simulink model "AccelCtrl_ACC_test"  (R2019b)
settings: Solver=FixedStepAuto  StartTime=0.0  StopTime=inf  FixedStep=0.001  RelTol=1e-3  EnableMultiTasking=on
libraries: CarMaker4SL x42, simulink x3
(part 3 of 3)

== matlab function AccelCtrl_ACC_test/CarMaker/VehicleControl/AccelCtrl/ACC ECU/MATLAB Function ==
  data: v_f input; s_of_t output size=400; a_f input; dist input; v_ego input; a_ego input; KJ input; KT input; KDS input; KJV input; KTV input; KDSV input; speed_limit input; MAX_ACC input; MIN_ACC input; v_of_t output size=400; t_data output size=400; a_des output; cost_optimal output; SET_SPEED input
% clc
% clear all
% close all
% 
% 
% v_f = 10;
% a_f = 0;
% dist = 20;
% v_ego = 7;
% a_ego = 0;
% KJ = 1;
% KT = 1;
% KDS = 10;
% speed_limit= 20;
% MAX_ACC = 2;
% MIN_ACC = -3;
% 
% 
% [s_of_t, v_of_t,t_data] = acc_planning(v_f,a_f,dist,v_ego,a_ego,KJ,KT,KDS,speed_limit,MAX_ACC, MIN_ACC);
% 
% 
% figure
% plot(t_data,s_of_t,'-b')
% title("s of t")
% 
% figure
% plot(t_data,v_of_t,'-b')
% title("v of t")

function [s_of_t, v_of_t,t_data,a_des,cost_optimal] = acc_planning(v_f,a_f,dist,v_ego,a_ego,KJ,KT,KDS,KJV, KTV, KDSV,...
    speed_limit,MAX_ACC, MIN_ACC,SET_SPEED)

    DT = 1 ; % Delta T [s]
    MAXT = 5;% [s]
    MINT = 2; % [s]
    MINT_V = 2;
    MAXT_V = 10;
    
    
    DS = 0.5;
    DV = 0.5;
    
    D0 = 5;
    TTC = 3;
    s_of_t = zeros(200,1);
    v_of_t = zeros(200,1);
    t_data = zeros(200,1); 
    a_des = 0;
    cost_optimal = zeros(1,12);
    
    if dist > 100
        [cost_graph] = cal_velocity_control(MINT_V,DT,MAXT_V, SET_SPEED,DV,v_ego, a_ego,KJV, KTV, KDSV);
        [cost_optimal] = check_quantic_status(cost_graph,speed_limit, MAX_ACC, MIN_ACC);
        [s_of_t, v_of_t,t_data] = combination_quantic(cost_optimal);
        a_des = PID_control_a(v_of_t,v_ego);
   
        
    elseif dist > 0 && dist < 100
        
        cost_graph = cal_distance_control(MINT,DT,MAXT,v_f,a_f,dist,D0,TTC,DS,v_ego,a_ego,KJ,KT,KDS)
        cost_optimal = check_status(cost_graph,speed_limit, MAX_ACC, MIN_ACC);
        [s_of_t, v_of_t,t_data] = combination(cost_optimal);
        a_des = PID_control_a(v_of_t,v_ego);
    end
end


function a_des = PID_control_a(v_of_t,v_ego)
    a_des = 0.2 * (v_of_t(2) - v_ego);
end

function v_des = PID_control_v(v_of_t,v_ego)
    v_des = 1 * (v_of_t(2) - v_ego);
end


function v_f_t = cal_v_f_t(v_f, a_f, Ti)
    %calculate v_f of time.
    v_f_t = v_f + a_f * Ti;
end
    

function dist_t = cal_dist_t(dist,v_f,a_f,Ti)
    %calculate distance of time.
    dist_t = dist + v_f * Ti + 1/2 * a_f * Ti^2;
end


function [s_des] = cal_s_des(D0, TTC, v_f_t)
    %calculate desired s.
    s_des = D0 + TTC * v_f_t;
end


function [s_target] = cal_s_target(s_des,dist_t)
    %calculate s target.
    s_target = dist_t - s_des;
end

function [s_target_d] = cal_s_target_d(v_f_t, TTC, a_f)
    %calculate v_f of time.
    s_target_d = v_f_t - TTC * a_f;
end


function [s_target_dd] = cal_s_target_dd(a_f)
    s_target_dd = a_f;
end

function [cost_graph] = cal_distance_control(MINT,DT,MAXT,v_f,a_f,dist,D0,TTC,DS,v_ego,a_ego,KJ,KT,KDS)
    
    cost_graph = ones(400,12)* 500; 
    index = 1;
    for Ti = MINT : DT : MAXT
        v_f_t = cal_v_f_t(v_f, a_f, Ti);
        dist_t = cal_dist_t(dist,v_f,a_f,Ti);
        [s_des] = cal_s_des(D0, TTC, v_f_t);
        [s_target] = cal_s_target(s_des,dist_t);
        [s_target_d] = cal_s_target_d(v_f_t, TTC, a_f);
        [s_target_dd] = cal_s_target_dd(a_f);
        delta_s = 0.1 * s_target;
        
        for Si = (s_target - delta_s) : DS : (s_target + delta_s) 
            s0 = 0;
            v0 = v_ego;
            a0 = a_ego;
            se = Si;
            ve = s_target_d;
            ae = s_target_dd;
            [a0, a1, a2, a3, a4,a5] = quintic_polynomial(s0, ...
                v0, a0, se, ve, ae,Ti);
            %get the quintic polu parameters;
            [jerk] = cal_jerk(a3,a4,a5,Ti);
            cost_J = mean(abs(jerk));
            cost_T = Ti;
            cost_DS = sqrt((s_target - Si)^2);
            cost_total = KJ * cost_J + KT * cost_T + KDS * cost_DS;
            cost_graph(index,:) = [cost_total,Ti,Si,cost_J,cost_T,cost_DS,...
                a0, a1, a2, a3, a4, a5];
            
            index = index + 1;
        end
    end
    cost_graph = sortrows(cost_graph);
end

function [cost_graph] = cal_velocity_control(MINT_V,DT,MAXT_V, SET_SPEED,DV,v_ego, a_ego,KJV, KTV, KDSV)
    cost_graph = ones(400,11)* 500;    
    index = 1;
    delta_v = 0.1 * SET_SPEED;

    for Ti = MINT_V : DT : MAXT_V
        for Ve = SET_SPEED - delta_v : DV : SET_SPEED + delta_v 
            s0 = 0;
            v0 = v_ego;
            a0 = a_ego;
            ve = Ve;
            ae = 0;
            [a0, a1, a2, a3, a4] = quantic_polynomial(s0, ...
                v0, a0, ve, ae,Ti)
            [jerk] = cal_quantic_jerk(a3,a4,Ti);
            cost_J = mean(abs(jerk));
            cost_T = Ti;
            cost_DV = sqrt((SET_SPEED - Ve)^2);
            cost_total = KJV * cost_J + KTV * cost_T + KDSV * cost_DV;
            cost_graph(index,:) = [cost_total,Ti,Ve,cost_J,cost_T,cost_DV,...
                a0, a1, a2, a3, a4];

            index = index + 1;
        end
    end
        cost_graph = sortrows(cost_graph);
end


function [cost_optimal] = check_status(cost_graph,speed_limit, MAX_ACC, MIN_ACC)
    i = 1;
    COND = 1;
    cost_optimal = zeros(1,12);
    if isempty(cost_graph)
        cost_optimal=  zeros(1,12);
        fprintf("error in cost graph.");
        return;
    end
    
    
    
    while COND == 1
         
        vt = [];
        at = [];
        
        
        poly_para = cost_graph(i,7:12);
        a0 = poly_para(1); a1 = poly_para(2); a2 = poly_para(3); 
        a3 = poly_para(4); a4 = poly_para(5); a5 = poly_para(6);
        
        Te = cost_graph(i,2);
        
        
        
        for t = 0:0.5:Te
            vt = [vt, calc_first_derivative(a1,a2,a3,a4,a5,t)];
            at = [at, calc_second_derivative(a2,a3,a4,a5,t)];
        end
        
        if (max(abs(vt)) <= speed_limit && max(at) <= MAX_ACC && min(at) >= MIN_ACC)
            cost_optimal = cost_graph(i,:);
            COND = 2;
        end
        
        i = i + 1;
        
        if i > size(cost_graph,1)
            COND = 2;
            cost_optimal  = cost_graph(1,:);
        end
    end
end

function [cost_optimal] = check_quantic_status(cost_graph,speed_limit, MAX_ACC, MIN_ACC)
    i = 1;
    COND = 1;
    cost_optimal = zeros(1,12);
    if isempty(cost_graph)
        cost_optimal=  zeros(1,12);
        fprintf("error in cost graph.");
        return;
    end
    
  
    while COND == 1
         
        vt = [];
        at = [];
        
        
        poly_para = cost_graph(i,7:11);
        a0 = poly_para(1); a1 = poly_para(2); a2 = poly_para(3); 
        a3 = poly_para(4); a4 = poly_para(5); 
        
        Te = cost_graph(i,2);
        
        
        
        for t = 0:0.5:Te
            vt = [vt, calc_quantic_first_derivative(a1,a2,a3,a4,t)];
            at = [at, calc_quantic_second_derivative(a2,a3,a4,t)];
        end
        
        if (max(abs(vt)) <= speed_limit && max(at) <= MAX_ACC && min(at) >= MIN_ACC)
            cost_optimal = cost_graph(i,:);
            COND = 2;
        end
        
        i = i + 1;
        
        if i > size(cost_graph,1)
            COND = 2;
            cost_optimal  = cost_graph(1,:);
        end
    end
end


function [s_of_t, v_of_t,t_data] = combination(cost_optimal)
    if isempty(cost_optimal)
       s_of_t = zeros(200,1);
        v_of_t = zeros(200,1);
        t_data = zeros(200,1);
        fprintf("error in optimal cost graph.");
        return;
    end

    Te = cost_optimal(2);
    poly_para = cost_optimal(7:12);
    a0 = poly_para(1); a1 = poly_para(2); a2 = poly_para(3); 
    a3 = poly_para(4); a4 = poly_para(5); a5 = poly_para(6);
    s_of_t = zeros(200,1);
    v_of_t = zeros(200,1);
    t_data = zeros(200,1);
    
    for t = 0 : 0.1 : Te
        s_of_t = [s_of_t,calc_point(a0,a1,a2,a3,a4,a5,t)];
        v_of_t = [v_of_t,calc_first_derivative(a1,a2,a3,a4,a5,t)];
        t_data = [t_data,t];
    end
end

function [s_of_t, v_of_t,t_data] = combination_quantic(cost_optimal)
    if isempty(cost_optimal)
        s_of_t = zeros(200,1);
        v_of_t = zeros(200,1);
        t_data = zeros(200,1);
        fprintf("error in optimal cost graph.");
        return;
    end

    Te = cost_optimal(2);
    poly_para = cost_optimal(7:11);
    a0 = poly_para(1); a1 = poly_para(2); a2 = poly_para(3); 
    a3 = poly_para(4); a4 = poly_para(5); 
    s_of_t = zeros(200,1);
    v_of_t = zeros(200,1);
    t_data = zeros(200,1);
    for t = 0 : 0.1 : Te
        s_of_t = [s_of_t,cal_quantic_point(a0,a1,a2,a3,a4,t)];
        v_of_t = [v_of_t,calc_quantic_first_derivative(a1,a2,a3,a4,t)];
        t_data = [t_data,t];
    end
end


function [xt] = calc_point(a0,a1,a2,a3,a4,a5,t)
xt = a0 + a1 * t + a2 * t ^2 + a3 * t^3 + a4 * t^4+a5 * t^5;
end

function [xt] = cal_quantic_point(a0,a1,a2,a3,a4,T)
    xt = a0 + a1 * T + a2 * T^2 + a3 * T^3 + a4 * T^4;
end

function [xt] =calc_first_derivative(a1,a2,a3,a4,a5,t)
xt = a1 + 2 * a2 * t + 3 * a3 * t^2 + 4 * a4 * t^3  +  5 * a5 * t^4;
end

function [xt] =calc_quantic_first_derivative(a1,a2,a3,a4,t)
xt = a1 + 2 * a2 * t + 3 * a3 * t^2 + 4 * a4 * t^3;
end


function [xt]  = calc_second_derivative(a2,a3,a4,a5,t)
xt = 2* a2 + 6* a3 * t + 12 * a4 * t^2 + 20* a5 *t^3;
end

function [xt]  = calc_quantic_second_derivative(a2,a3,a4,t)
xt = 2* a2 + 6* a3 * t + 12 * a4 * t^2;
end

function [xt] = calc_third_derivative(a3,a4,a5,t)
xt =6 * a3 + 24 * a4 * t + a5 * t^2;
end

function [jerk] = cal_jerk(a3,a4,a5,Ti)
    jerk = [];
    for i = 0:0.1:Ti
        jerk = [jerk,  6* a3  + 24 * a4 * i + 60* a5 *i^2];
    end
end

function [jerk] = cal_quantic_jerk(a3,a4,Ti)
    jerk = [];
    for i = 0:0.1:Ti
        jerk = [jerk,  6* a3 + 24 * a4 * i];
    end
end

function [a0, a1, a2, a3, a4,a5] = quintic_polynomial(xs, ...
    vxs, axs, xe, vxe, axe,T)
% A = [0,0,0,0,0,1; T^5,T^4,T^3,T^2,T,1;...
%     0,0,0,0,1,0 ; 5*T^4  4*T^3 3*T^2 2*T 1 0 ; ...
%     0 0 0 2 0 0; 20*T^3 12*T^2 6*T 2 0 0];
% b = [xs, xe, vxs, vxe, axs, 0]';
% x = A\b;
% a5 = x(1);
% a4 = x(2);
% a3 = x(3);
% a2 = x(4);
% a1 = x(5);
% a0 = x(6);
A = [T^3 T^4 T^5; 3*T^2 4*T^3 5*T^4; 6*T 12*T^2 20*T^3];
b = [(xe - xs  - vxs*T - 0.5*axs*T^2); (vxe- vxs - axs*T ); (axe - axs)];

if det(A) == 0
    a0 = [];
    a1 = [];
    a2 = [];

    a3 = [];
    a4 = [];
    a5 = [];  
    
    fprintf('cannot calculate quintic polynomial paras.');
    return;
end


    
    
x = pinv(A) * b;
a0 = xs;
a1 = vxs;
a2 = axs/2;

a3 = x(1);
a4 = x(2);
a5 = x(3);
end

function [a0, a1, a2, a3, a4] = quantic_polynomial(xs, ...
    vxs, axs, vxe, axe,T)
    
    A  =[1,0,0,0,0;0,1,0,0,0;0,0,2,0,0;...
        0,1,2*T,3*T^2,4*T^3;0,0,2,6*T,12*T^2];
    
    if det(A) == 0
        a0 = [];
        a1 = [];
        a2 = [];

        a3 = [];
        a4 = [];


        fprintf('cannot calculate quintic polynomial paras.');
        return;
    end
    
    
    b = [xs,vxs,axs,vxe,axe]';
    x = pinv(A) * b;
    
    a0 = x(1);
    a1 = x(2);
    a2 = x(3);
    a3 = x(4);
    a4 = x(5);
end

== matlab function AccelCtrl_ACC_test/CarMaker/VehicleControl/AccelCtrl/ACC ECU/Subsystem/MATLAB Function ==
  data: ACC_MODE input; v_des output; a_des output; traf_sign input; velocity input; dist input; time input; CONST_LIMIT input; dist output; v_des_pre input; case_num output

% clc
% clear all
% close all
% traf_sign = 0;
% velocity = 30;
% dist = 100;
% time = 12;
% CONST_LIMIT = 40;
% ACC_MODE = 0;

function [v_des,a_des,dist,case_num] = intesec_cross(ACC_MODE, traf_sign, velocity, dist, time,CONST_LIMIT,v_des_pre)  
%% this is a function that provide desired velocity, and distance to traffic light;
    % input: trafic_sign with green = 0; red = 1; yellow = 2;
    %        velocity in unit of kph;
    %        dist, and time is distance(m) to cross, and traffic time left
    %        CONST_LIMIT is velocity limit at cross, which is a reference CONSTANT velocity from
    %        ACC module.
    %        v_des_pre preseve previous v_des for next step use.
    
    % output: desired velocity for ACC module, in unit of kph;
    %         dist is distance(m) to front cross;
    
    green = 0;
    red = 1;
    yellow = 2;
    v = velocity / 3.6;
    distance = dist;
    CONST_LIMIT = CONST_LIMIT / 3.6;
    delta_t = 0.5;
    v_des = 0;
    a_des = 0;
    
    
    switch traf_sign
        case green
            if ACC_MODE == 0
                T = time;
                a = 2 * (dist - v * T) / (T^2 + 0.0001);
                v_temp = v + a * T;

                if (a >= 1) || ((a >= 0) && (a < 1) && (v_temp >= CONST_LIMIT))
                    v_des = 0;
                    a_des = 0;
                    case_num = 1;
                    
                elseif ((a < 0) && (v_temp >= 0) && (v_temp <= CONST_LIMIT))
                    v_des = CONST_LIMIT;
                    a_des = 0;
                    case_num = 2;
                else
                    v_des = v + a * T;
                    a_des = a;
                    case_num = 3;
                end
                
            else %(ACC_MODE == 1)
                T_ACC = dist / (v + 0.0001);
                if T_ACC < time - delta_t
                    v_des = v;
                    a_des = 0;
                    case_num = 4;
                    
                elseif T_ACC > time + delta_t
                    v_des = 0;
                    a_des = 0;
                    case_num = 5;
                    
                else
                    v_des = v_des_pre;
                    a_des = 0;
                    case_num = 6;
                end
            end
                          
        case red
            T = time + 1;
            a = 2 * (dist - v * T) / T^2;
            v_temp = v + a * T;
            
            
            if (a < -1)
                v_des = 0;
                a_des = 0;
                case_num = 7;
                
            elseif (a <=0 && a>= -1)
                v_des = v_temp;
                a_des = a;
                case_num = 8;
                
            elseif (a >= 0 && a <= 1 && v_temp < CONST_LIMIT)
                v_des = v_temp ; 
                a_des = a;
                case_num = 9;
                
            else
                v_des = CONST_LIMIT;
                a_des = 0;
                case_num = 10;
            end
       
    
                
        otherwise
            v_des = 0;
            a_des = 0;
            case_num = 11;
            
            
    end
    
    
    
    end
